simulink model "controlPunto2"  (R2024b)
settings: Solver=ode45  StartTime=0.0  StopTime=20  RelTol=1e-3
settings Model: Creator=juanp  LastModifiedBy=juanp

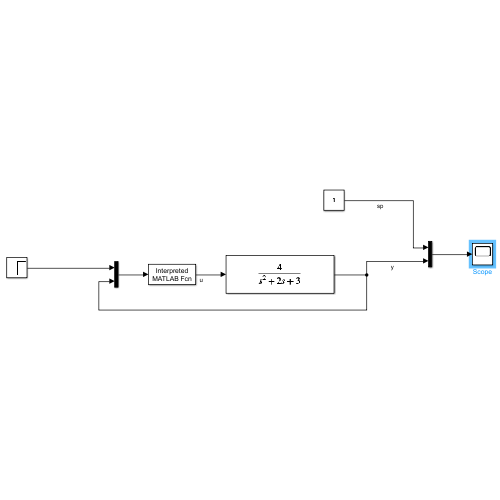
[thumbnail: Simulink's stored preview of the top-level diagram]
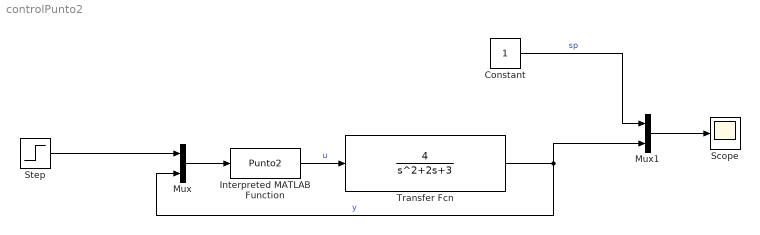
== system controlPunto2 ==
  Constant : Constant
  Interpreted MATLAB Function : MATLABFcn  MATLABFcn=Punto2
  Mux : Mux  Inputs=2
  Mux1 : Mux  Inputs=2
  Scope : Scope
  Step : Step  SampleTime=0
  Transfer Fcn : TransferFcn  Numerator=[4]  Denominator=[1 2 3]
  wires:
  Transfer Fcn/1 -> Mux1/2, Mux/2  "y"
  Interpreted MATLAB Function/1 -> Transfer Fcn/1  "u"
  Step/1 -> Mux/1
  Mux/1 -> Interpreted MATLAB Function/1
  Mux1/1 -> Scope/1
  Constant/1 -> Mux1/1  "sp"
